simulink model "lpfbuttter2nd"  (R2024b)
settings: Solver=ode4  StartTime=0.0  StopTime=2  FixedStep=1e-3  RelTol=1e-3
libraries: simulink x1, cstblocks x1
settings Model: Creator=auralius  LastModifiedBy=auralius

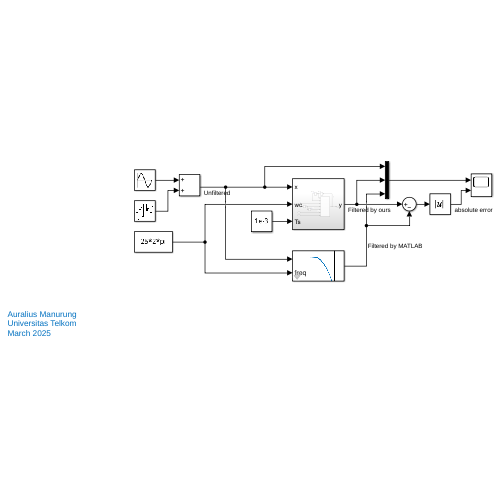
[thumbnail: Simulink's stored preview of the top-level diagram]
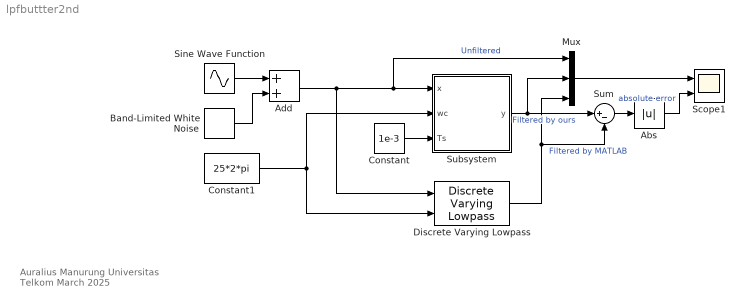
== system lpfbuttter2nd ==
  note: Auralius Manurung
      | Universitas Telkom
      | March 2025
  Abs : Abs  SaturateOnIntegerOverflow=off
  Add : Sum
  Band-Limited White Noise : simulink/Sources/Band-Limited White Noise  Cov=[0.1]  Ts=1e-3  seed=[23341]
  Constant : Constant  Value=1e-3
  Constant1 : Constant  Value=25*2*pi
  Discrete Varying Lowpass : cstblocks/Linear Parameter Varying/Discrete Varying Lowpass  N=2  w0=0  Ts=1e-3
  Mux : Mux  Inputs=3
  Scope1 : Scope  NumInputPorts=2
  Sine Wave Function : Sin  Frequency=50*pi  SampleTime=0
  Subsystem : Subsystem
  Sum : Sum  Inputs=|+-
  wires:
  Constant/1 -> Subsystem/3(Ts)
  Sine Wave Function/1 -> Add/1
  Band-Limited White Noise/1 -> Add/2
  Constant1/1 -> Subsystem/2(wc), Discrete Varying Lowpass/2
  Add/1 -> Discrete Varying Lowpass/1, Mux/1, Subsystem/1(x)  "Unfiltered"
  Subsystem/1(y) -> Sum/1, Mux/2  "Filtered by ours"
  Discrete Varying Lowpass/1 -> Mux/3, Sum/2  "Filtered by MATLAB"
  Sum/1 -> Abs/1
  Abs/1 -> Scope1/2  "absolute error"
  Mux/1 -> Scope1/1

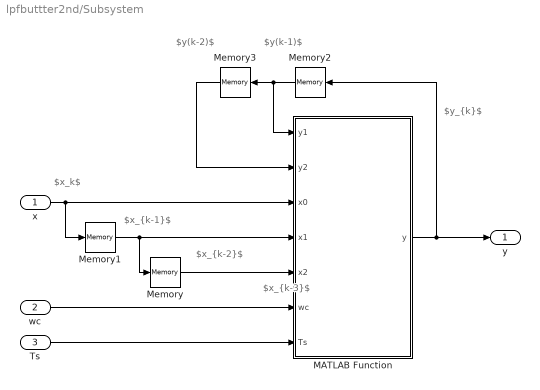
== system lpfbuttter2nd/Subsystem ==
  note: $x_k$
  note: $x_{k-2}$
  note: $x_{k-1}$
  note: $y_{k}$
  note: $y(k-2)$
  note: $y(k-1)$
  note: $x_{k-3}$
  x : Inport
  wc : Inport  Port=2
  Ts : Inport  Port=3
  MATLAB Function : MATLAB Function  TreatAsAtomicUnit=on
  Memory{,1..3} (4 alike) : Memory  InheritSampleTime=on
  y : Outport
  wires:
  wc/1 -> MATLAB Function/6(wc)
  MATLAB Function/1(y) -> y/1, Memory2/1
  Memory2/1 -> MATLAB Function/1(y1), Memory3/1
  Ts/1 -> MATLAB Function/7(Ts)
  Memory1/1 -> MATLAB Function/4(x1), Memory/1
  Memory/1 -> MATLAB Function/5(x2)
  x/1 -> Memory1/1, MATLAB Function/3(x0)
  Memory3/1 -> MATLAB Function/2(y2)

== matlab function lpfbuttter2nd/Subsystem/MATLAB Function ==
  data: y1 input; y2 input; x0 input; x1 input; x2 input; y output; wc input; Ts input
function y = LPF(y1, y2, x0, x1, x2, wc, Ts)
% y1 is y(k-1)
% y2 is y(k-2)
% x0 is x(k)
% x1 is x(k-1)
% x2 is x(k-2)

sq22 = 2*sqrt(2);
Tswc = Ts * wc;
A = 1 + sq22/Tswc + 4/Tswc^2;
B = 2 - 8/Tswc^2;  
C = 1 - sq22/Tswc + 4/Tswc^2;

y = (x0 + 2*x1 + x2 - y1*B - y2*C ) / A;
